simulink library "HY_General_Library"  (R2018b)
settings: Solver=ode45  StartTime=0.0  StopTime=10.0  RelTol=1e-3  EnableMultiTasking=on
undefined symbols (not defined in the file or in its folder): dT, Slope1, Slope2
libraries: simulink x63, $bdroot x4
(part 3 of 5)

== system HY_General_Library/Hysteresis_Blocks/HysteresisB ==
  OFF : Inport
  u : Inport  Port=2
  ON : Inport  Port=3
  RESET : Constant  Value=0  OutDataTypeStr=boolean
      settings: AttributesFormatString=%<OutDataTypeStr>
  Relational Operator : RelationalOperator  Operator=>  OutDataTypeStr=boolean  RndMeth=Nearest
  Relational Operator1 : RelationalOperator  Operator=<=  OutDataTypeStr=boolean  RndMeth=Nearest
  SET : Constant  OutDataTypeStr=boolean
      settings: AttributesFormatString=%<OutDataTypeStr>
  Switch : Switch  Criteria=u2 ~= 0  SaturateOnIntegerOverflow=on
  Switch1 : Switch  Criteria=u2 ~= 0  SaturateOnIntegerOverflow=on
  Unit Delay : UnitDelay  InitialCondition=InitialValue  SampleTime=-1
      settings: AttributesFormatString=Init: %<X0>
  y : Outport
  wires:
  RESET/1 -> Switch/1
  SET/1 -> Switch1/1
  Relational Operator/1 -> Switch/2
  Relational Operator1/1 -> Switch1/2
  Switch1/1 -> Switch/3
  Unit Delay/1 -> Switch1/3
  Switch/1 -> y/1, Unit Delay/1
  ON/1 -> Relational Operator1/2
  u/1 -> Relational Operator/1, Relational Operator1/1
  OFF/1 -> Relational Operator/2

== system HY_General_Library/Limit_Blocks/GrandientLimiter ==
  TargetValue : Inport  RequirementInfo={} %GIDa_f6d18a4e_084c_45e5_9882_4c3ecc41a03a
  BaseValue : Inport  RequirementInfo={} %GIDa_fa325680_5d49_4650_9e93_54c2fe60e26b  Port=2
  Reset : Inport  Port=3  OutDataTypeStr=boolean
  ResetValue : Inport  Port=4
  GrdtPos : Inport  RequirementInfo={} %GIDa_5e77dc31_cedd_4c5f_966e_ba8c10611931  Port=5
  GrdtNeg : Inport  RequirementInfo={} %GIDa_da933117_8913_4446_8ae4_767cc6412277  Port=6
  SampleTime : Inport  RequirementInfo={} %GIDa_02549e31_b069_4371_b83e_0eb5bce206e9  Port=7
  Abs1 : Abs
  Abs2 : Abs
  Gain1 : Gain  Gain=-1
  MinMax1 : MinMax  Function=max  Inputs=2
  MinMax2 : MinMax  Inputs=2
  Product : Product
  Product1 : Product
  Subtract : Sum  Inputs=+-
  Subtract1 : Sum
  Switch : Switch  Criteria=u2 ~= 0  SaturateOnIntegerOverflow=on
  GrdtLimdValue : Outport  RequirementInfo={} %GIDa_7967a4c3_b106_4517_b83e_55608d1226d7
  wires:
  MinMax2/1 -> MinMax1/2
  Gain1/1 -> MinMax1/1
  Abs2/1 -> Product/1
  MinMax1/1 -> Subtract1/1
  TargetValue/1 -> Subtract/1
  Abs1/1 -> Product1/2
  Product/1 -> Gain1/1
  SampleTime/1 -> Product1/1, Product/2
  Subtract/1 -> MinMax2/2
  Subtract1/1 -> Switch/3
  BaseValue/1 -> Subtract/2, Subtract1/2
  Product1/1 -> MinMax2/1
  GrdtPos/1 -> Abs1/1
  GrdtNeg/1 -> Abs2/1
  ResetValue/1 -> Switch/1
  Reset/1 -> Switch/2
  Switch/1 -> GrdtLimdValue/1

== system HY_General_Library/Limit_Blocks/LIMIT ==
  Max : Inport
  u : Inport  Port=2
  Min : Inport  Port=3
  Data Type Propagation : simulink/Signal Attributes/Data Type Propagation  PropDataType=fixdt(1, 16)  IfRefDouble=double  IfRefSingle=single  IsSigned=IsSigned1  NumBitsBase=NumBits1  NumBitsMult=1  NumBitsAdd=0  NumBitsAllowFinal=1:128  PropScaling=2^-10  ValuesUsedBestPrec=[5 -7]  SlopeBase=min([Slope1 Slope2])  SlopeMult=1  SlopeAdd=0  BiasBase=Bias1  BiasMult=1  BiasAdd=0
      settings: SourceProductName=Simulink  SourceProductBaseCode=SL
  Data Type Propagation1 : simulink/Signal Attributes/Data Type Propagation  PropDataType=fixdt(1, 16)  IfRefDouble=double  IfRefSingle=single  IsSigned=IsSigned1  NumBitsBase=NumBits1  NumBitsMult=1  NumBitsAdd=0  NumBitsAllowFinal=1:128  PropScaling=2^-10  ValuesUsedBestPrec=[5 -7]  SlopeBase=min([Slope1 Slope2])  SlopeMult=1  SlopeAdd=0  BiasBase=Bias1  BiasMult=1  BiasAdd=0
      settings: SourceProductName=Simulink  SourceProductBaseCode=SL
  MinMax : MinMax  Inputs=2  SaturateOnIntegerOverflow=on  InputSameDT=on
  MinMax1 : MinMax  Function=max  Inputs=2  OutDataTypeStr=Inherit: Inherit via back propagation  SaturateOnIntegerOverflow=on
  y : Outport  InitialOutput=0
  wires:
  MinMax/1 -> y/1, Data Type Propagation1/3
  MinMax1/1 -> MinMax/2, Data Type Propagation/3
  Min/1 -> MinMax1/2
  u/1 -> Data Type Propagation/2, Data Type Propagation/1, Data Type Propagation1/2, Data Type Propagation1/1, MinMax1/1
  Max/1 -> MinMax/1

== system HY_General_Library/Limit_Blocks/Limit_Flag ==
  Max : Inport
  u : Inport  Port=2
  Min : Inport  Port=3
  Data Type Propagation : simulink/Signal Attributes/Data Type Propagation  PropDataType=fixdt(1, 16)  IfRefDouble=double  IfRefSingle=single  IsSigned=IsSigned1  NumBitsBase=NumBits1  NumBitsMult=1  NumBitsAdd=0  NumBitsAllowFinal=1:128  PropScaling=2^-10  ValuesUsedBestPrec=[5 -7]  SlopeBase=min([Slope1 Slope2])  SlopeMult=1  SlopeAdd=0  BiasBase=Bias1  BiasMult=1  BiasAdd=0
      settings: SourceProductName=Simulink  SourceProductBaseCode=SL
  Data Type Propagation1 : simulink/Signal Attributes/Data Type Propagation  PropDataType=fixdt(1, 16)  IfRefDouble=double  IfRefSingle=single  IsSigned=IsSigned1  NumBitsBase=NumBits1  NumBitsMult=1  NumBitsAdd=0  NumBitsAllowFinal=1:128  PropScaling=2^-10  ValuesUsedBestPrec=[5 -7]  SlopeBase=min([Slope1 Slope2])  SlopeMult=1  SlopeAdd=0  BiasBase=Bias1  BiasMult=1  BiasAdd=0
      settings: SourceProductName=Simulink  SourceProductBaseCode=SL
  Logical Operator : Logic  OutDataTypeStr=boolean
  Logical Operator1 : Logic  Operator=NOT  Inputs=1  OutDataTypeStr=boolean
  MinMax : MinMax  Inputs=2  SaturateOnIntegerOverflow=on  InputSameDT=on
  MinMax1 : MinMax  Function=max  Inputs=2  OutDataTypeStr=Inherit: Inherit via back propagation  SaturateOnIntegerOverflow=on
  Relational Operator : RelationalOperator  Operator=>  OutDataTypeStr=boolean  RndMeth=Simplest  InputSameDT=on
  Relational Operator1 : RelationalOperator  Operator=<  OutDataTypeStr=boolean  RndMeth=Simplest  InputSameDT=on
  y : Outport  InitialOutput=0
  bMax : Outport  Port=2  InitialOutput=0
  bMin : Outport  Port=3  InitialOutput=0
  wires:
  Max/1 -> Relational Operator/2, MinMax/1
  u/1 -> MinMax1/1, Data Type Propagation1/1, Data Type Propagation1/2, Relational Operator1/1, Relational Operator/1, Data Type Propagation/2, Data Type Propagation/1
  Min/1 -> Relational Operator1/2, MinMax1/2
  MinMax1/1 -> Data Type Propagation/3, MinMax/2
  MinMax/1 -> Data Type Propagation1/3, y/1
  Logical Operator1/1 -> Logical Operator/1
  Relational Operator/1 -> Logical Operator1/1, bMax/1
  Logical Operator/1 -> bMin/1
  Relational Operator1/1 -> Logical Operator/2

== system HY_General_Library/Limit_Blocks/RateLimit_R ==
  u : Inport  RequirementInfo={} %GIDa_f6d18a4e_084c_45e5_9882_4c3ecc41a03a
  GrdtPos : Inport  RequirementInfo={} %GIDa_5e77dc31_cedd_4c5f_966e_ba8c10611931  Port=2
  GrdtNeg : Inport  RequirementInfo={} %GIDa_da933117_8913_4446_8ae4_767cc6412277  Port=3
  Reset : Inport  Port=4  OutDataTypeStr=boolean
  ResetVaule : Inport  Port=5
  dT : Inport  RequirementInfo={} %GIDa_02549e31_b069_4371_b83e_0eb5bce206e9  Port=6
  Constant : Constant  Value=0  OutDataTypeStr=boolean
      settings: AttributesFormatString=%<OutDataTypeStr>
  Constant1 : Constant  Value=0  OutDataTypeStr=Inherit: Inherit via back propagation
      settings: AttributesFormatString=%<OutDataTypeStr>
  Constant2 : Constant  Value=0  OutDataTypeStr=Inherit: Inherit via back propagation
      settings: AttributesFormatString=%<OutDataTypeStr>
  MinMax1 : MinMax  Function=max  Inputs=2  InputSameDT=on
  MinMax2 : MinMax  Inputs=2  InputSameDT=on
  MinMax3 : MinMax  Inputs=2  InputSameDT=on
  MinMax4 : MinMax  Function=max  Inputs=2  InputSameDT=on
  Product : Product
  Product1 : Product
  Subtract : Sum  Inputs=+-
  Subtract1 : Sum
  Switch : Switch  Criteria=u2 ~= 0  SaturateOnIntegerOverflow=on
      settings: AttributesFormatString=|
      | %<Criteria>
      | Threshold=%<Threshold>
  Switch1 : Switch  Criteria=u2 ~= 0  SaturateOnIntegerOverflow=on
      settings: AttributesFormatString=|
      | %<Criteria>
      | Threshold=%<Threshold>
  Unit Delay : UnitDelay  InitialCondition=1  SampleTime=-1
      settings: AttributesFormatString=<Initial=%<InitialCondition>>
  Unit Delay1 : UnitDelay  SampleTime=-1
      settings: AttributesFormatString=<Initial=%<InitialCondition>>
  y : Outport  RequirementInfo={} %GIDa_7967a4c3_b106_4517_b83e_55608d1226d7
  wires:
  Switch/1 -> Unit Delay1/1, y/1
  Reset/1 -> Switch/2
  ResetVaule/1 -> Switch/1
  Product1/1 -> MinMax3/1
  Subtract1/1 -> Switch1/3
  Subtract/1 -> MinMax1/2
  dT/1 -> Product1/1, Product/2
  Product/1 -> MinMax4/1
  GrdtPos/1 -> Product/1
  u/1 -> [u], Subtract/1
  MinMax2/1 -> Subtract1/1
  GrdtNeg/1 -> Product1/2
  MinMax4/1 -> MinMax2/1
  MinMax1/1 -> MinMax2/2
  Switch1/1 -> Switch/3
  Unit Delay/1 -> Switch1/2
  Constant/1 -> Unit Delay/1
  Unit Delay1/1 -> Subtract/2, Subtract1/2
  [u] -> Switch1/1
  Constant1/1 -> MinMax4/2
  Constant2/1 -> MinMax3/2
  MinMax3/1 -> MinMax1/1

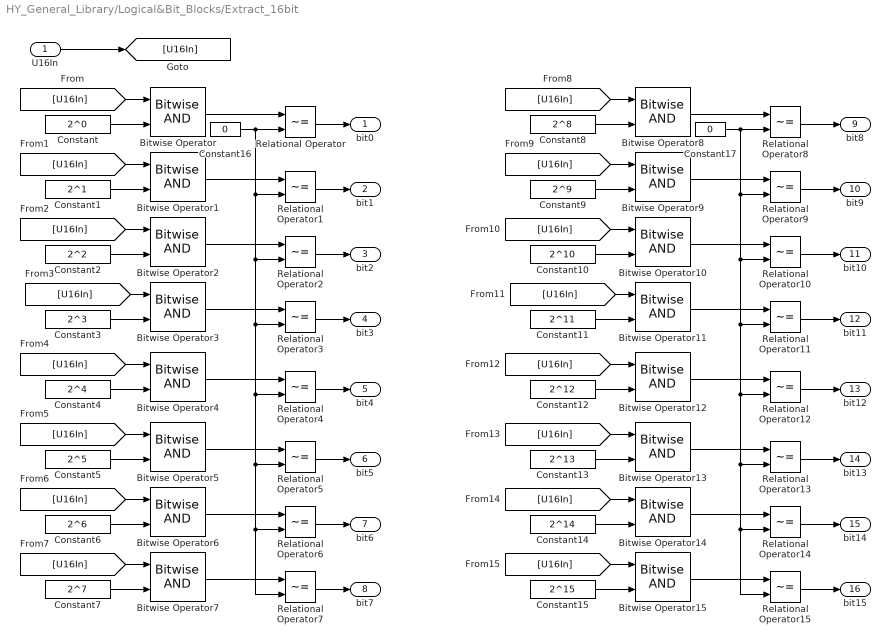
== system HY_General_Library/Logical&Bit_Blocks/Extract_16bit ==
  U16In : Inport
  Bitwise Operator{,1..15} (16 alike) : simulink/Logic and Bit Operations/Bitwise Operator  logicop=AND  UseBitMask=off  NumInputPorts=2  BitMask=bin2dec('11011001')  BitMaskRealWorld=Stored Integer
  Constant : Constant  Value=2^0  OutDataTypeStr=uint16
  Constant1 : Constant  Value=2^1  OutDataTypeStr=uint16
  Constant10 : Constant  Value=2^10  OutDataTypeStr=uint16
  Constant11 : Constant  Value=2^11  OutDataTypeStr=uint16
  Constant12 : Constant  Value=2^12  OutDataTypeStr=uint16
  Constant13 : Constant  Value=2^13  OutDataTypeStr=uint16
  Constant14 : Constant  Value=2^14  OutDataTypeStr=uint16
  Constant15 : Constant  Value=2^15  OutDataTypeStr=uint16
  Constant16 : Constant  Value=0  OutDataTypeStr=uint16
  Constant17 : Constant  Value=0  OutDataTypeStr=uint16
  Constant2 : Constant  Value=2^2  OutDataTypeStr=uint16
  Constant3 : Constant  Value=2^3  OutDataTypeStr=uint16
  Constant4 : Constant  Value=2^4  OutDataTypeStr=uint16
  Constant5 : Constant  Value=2^5  OutDataTypeStr=uint16
  Constant6 : Constant  Value=2^6  OutDataTypeStr=uint16
  Constant7 : Constant  Value=2^7  OutDataTypeStr=uint16
  Constant8 : Constant  Value=2^8  OutDataTypeStr=uint16
  Constant9 : Constant  Value=2^9  OutDataTypeStr=uint16
  Relational Operator{,1..15} (16 alike) : RelationalOperator  Operator=~=  OutDataTypeStr=boolean  RndMeth=Nearest
  bit0 : Outport
  bit1 : Outport  Port=2
  bit2 : Outport  Port=3
  bit3 : Outport  Port=4
  bit4 : Outport  Port=5
  bit5 : Outport  Port=6
  bit6 : Outport  Port=7
  bit7 : Outport  Port=8
  bit8 : Outport  Port=9
  bit9 : Outport  Port=10
  bit10 : Outport  Port=11
  bit11 : Outport  Port=12
  bit12 : Outport  Port=13
  bit13 : Outport  Port=14
  bit14 : Outport  Port=15
  bit15 : Outport  Port=16
  wires:
  U16In/1 -> [U16In]
  [U16In] -> Bitwise Operator/1
  Constant/1 -> Bitwise Operator/2
  [U16In] -> Bitwise Operator1/1
  Constant1/1 -> Bitwise Operator1/2
  [U16In] -> Bitwise Operator2/1
  Constant2/1 -> Bitwise Operator2/2
  [U16In] -> Bitwise Operator3/1
  Constant3/1 -> Bitwise Operator3/2
  [U16In] -> Bitwise Operator4/1
  Constant4/1 -> Bitwise Operator4/2
  [U16In] -> Bitwise Operator5/1
  Constant5/1 -> Bitwise Operator5/2
  [U16In] -> Bitwise Operator6/1
  Constant6/1 -> Bitwise Operator6/2
  [U16In] -> Bitwise Operator7/1
  Constant7/1 -> Bitwise Operator7/2
  Bitwise Operator1/1 -> Relational Operator1/1
  Bitwise Operator2/1 -> Relational Operator2/1
  Relational Operator2/1 -> bit2/1
  Relational Operator1/1 -> bit1/1
  Bitwise Operator3/1 -> Relational Operator3/1
  Relational Operator3/1 -> bit3/1
  Bitwise Operator4/1 -> Relational Operator4/1
  Relational Operator4/1 -> bit4/1
  Bitwise Operator5/1 -> Relational Operator5/1
  Relational Operator5/1 -> bit5/1
  Bitwise Operator6/1 -> Relational Operator6/1
  Relational Operator6/1 -> bit6/1
  Bitwise Operator7/1 -> Relational Operator7/1
  Relational Operator7/1 -> bit7/1
  [U16In] -> Bitwise Operator8/1
  Constant8/1 -> Bitwise Operator8/2
  [U16In] -> Bitwise Operator9/1
  Constant9/1 -> Bitwise Operator9/2
  [U16In] -> Bitwise Operator10/1
  Constant10/1 -> Bitwise Operator10/2
  [U16In] -> Bitwise Operator11/1
  Constant11/1 -> Bitwise Operator11/2
  [U16In] -> Bitwise Operator12/1
  Constant12/1 -> Bitwise Operator12/2
  [U16In] -> Bitwise Operator13/1
  Constant13/1 -> Bitwise Operator13/2
  [U16In] -> Bitwise Operator14/1
  Constant14/1 -> Bitwise Operator14/2
  [U16In] -> Bitwise Operator15/1
  Constant15/1 -> Bitwise Operator15/2
  Relational Operator10/1 -> bit10/1
  Relational Operator9/1 -> bit9/1
  Relational Operator8/1 -> bit8/1
  Relational Operator11/1 -> bit11/1
  Relational Operator12/1 -> bit12/1
  Relational Operator13/1 -> bit13/1
  Relational Operator14/1 -> bit14/1
  Relational Operator15/1 -> bit15/1
  Bitwise Operator/1 -> Relational Operator/1
  Relational Operator/1 -> bit0/1
  Constant16/1 -> Relational Operator1/2, Relational Operator2/2, Relational Operator3/2, Relational Operator4/2, Relational Operator5/2, Relational Operator7/2, Relational Operator6/2, Relational Operator/2
  Bitwise Operator9/1 -> Relational Operator9/1
  Bitwise Operator10/1 -> Relational Operator10/1
  Bitwise Operator11/1 -> Relational Operator11/1
  Bitwise Operator12/1 -> Relational Operator12/1
  Bitwise Operator13/1 -> Relational Operator13/1
  Bitwise Operator14/1 -> Relational Operator14/1
  Bitwise Operator15/1 -> Relational Operator15/1
  Bitwise Operator8/1 -> Relational Operator8/1
  Constant17/1 -> Relational Operator9/2, Relational Operator10/2, Relational Operator11/2, Relational Operator12/2, Relational Operator13/2, Relational Operator15/2, Relational Operator14/2, Relational Operator8/2

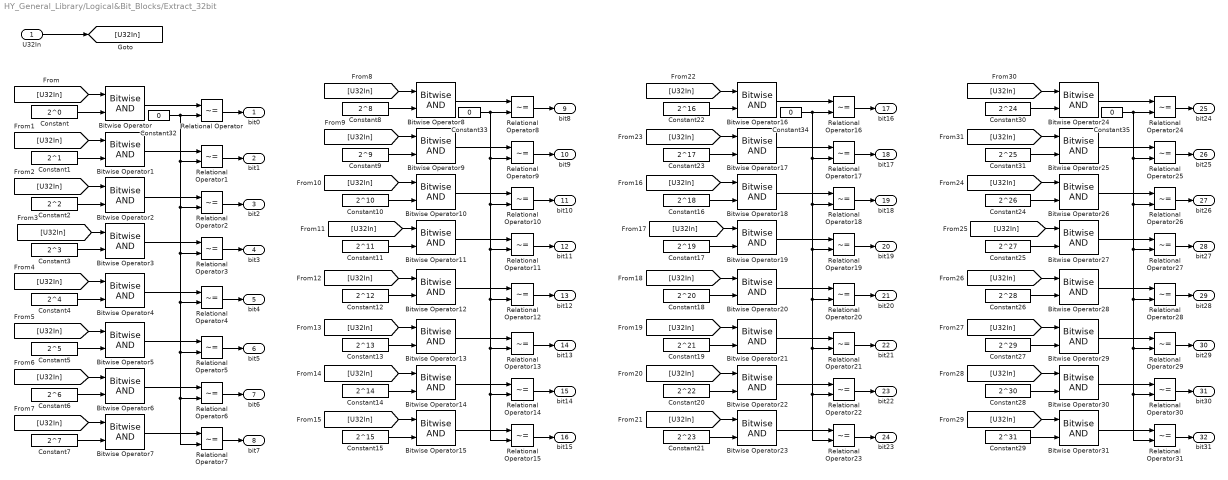
== system HY_General_Library/Logical&Bit_Blocks/Extract_32bit ==
  U32In : Inport
  Bitwise Operator{,1..31} (32 alike) : simulink/Logic and Bit Operations/Bitwise Operator  logicop=AND  UseBitMask=off  NumInputPorts=2  BitMask=bin2dec('11011001')  BitMaskRealWorld=Stored Integer
  Constant : Constant  Value=2^0  OutDataTypeStr=uint32
  Constant1 : Constant  Value=2^1  OutDataTypeStr=uint32
  Constant10 : Constant  Value=2^10  OutDataTypeStr=uint32
  Constant11 : Constant  Value=2^11  OutDataTypeStr=uint32
  Constant12 : Constant  Value=2^12  OutDataTypeStr=uint32
  Constant13 : Constant  Value=2^13  OutDataTypeStr=uint32
  Constant14 : Constant  Value=2^14  OutDataTypeStr=uint32
  Constant15 : Constant  Value=2^15  OutDataTypeStr=uint32
  Constant16 : Constant  Value=2^18  OutDataTypeStr=uint32
  Constant17 : Constant  Value=2^19  OutDataTypeStr=uint32
  Constant18 : Constant  Value=2^20  OutDataTypeStr=uint32
  Constant19 : Constant  Value=2^21  OutDataTypeStr=uint32
  Constant2 : Constant  Value=2^2  OutDataTypeStr=uint32
  Constant20 : Constant  Value=2^22  OutDataTypeStr=uint32
  Constant21 : Constant  Value=2^23  OutDataTypeStr=uint32
  Constant22 : Constant  Value=2^16  OutDataTypeStr=uint32
  Constant23 : Constant  Value=2^17  OutDataTypeStr=uint32
  Constant24 : Constant  Value=2^26  OutDataTypeStr=uint32
  Constant25 : Constant  Value=2^27  OutDataTypeStr=uint32
  Constant26 : Constant  Value=2^28  OutDataTypeStr=uint32
  Constant27 : Constant  Value=2^29  OutDataTypeStr=uint32
  Constant28 : Constant  Value=2^30  OutDataTypeStr=uint32
  Constant29 : Constant  Value=2^31  OutDataTypeStr=uint32
  Constant3 : Constant  Value=2^3  OutDataTypeStr=uint32
  Constant30 : Constant  Value=2^24  OutDataTypeStr=uint32
  Constant31 : Constant  Value=2^25  OutDataTypeStr=uint32
  Constant{32..35} (4 alike) : Constant  Value=0  OutDataTypeStr=uint32
  Constant4 : Constant  Value=2^4  OutDataTypeStr=uint32
  Constant5 : Constant  Value=2^5  OutDataTypeStr=uint32
  Constant6 : Constant  Value=2^6  OutDataTypeStr=uint32
  Constant7 : Constant  Value=2^7  OutDataTypeStr=uint32
  Constant8 : Constant  Value=2^8  OutDataTypeStr=uint32
  Constant9 : Constant  Value=2^9  OutDataTypeStr=uint32
  Relational Operator{,1..31} (32 alike) : RelationalOperator  Operator=~=  OutDataTypeStr=boolean  RndMeth=Nearest
  bit0 : Outport
  bit1 : Outport  Port=2
  bit2 : Outport  Port=3
  bit3 : Outport  Port=4
  bit4 : Outport  Port=5
  bit5 : Outport  Port=6
  bit6 : Outport  Port=7
  bit7 : Outport  Port=8
  bit8 : Outport  Port=9
  bit9 : Outport  Port=10
  bit10 : Outport  Port=11
  bit11 : Outport  Port=12
  bit12 : Outport  Port=13
  bit13 : Outport  Port=14
  bit14 : Outport  Port=15
  bit15 : Outport  Port=16
  bit16 : Outport  Port=17
  bit17 : Outport  Port=18
  bit18 : Outport  Port=19
  bit19 : Outport  Port=20
  bit20 : Outport  Port=21
  bit21 : Outport  Port=22
  bit22 : Outport  Port=23
  bit23 : Outport  Port=24
  bit24 : Outport  Port=25
  bit25 : Outport  Port=26
  bit26 : Outport  Port=27
  bit27 : Outport  Port=28
  bit28 : Outport  Port=29
  bit29 : Outport  Port=30
  bit30 : Outport  Port=31
  bit31 : Outport  Port=32
  wires:
  U32In/1 -> [U32In]
  [U32In] -> Bitwise Operator/1
  Constant/1 -> Bitwise Operator/2
  [U32In] -> Bitwise Operator1/1
  Constant1/1 -> Bitwise Operator1/2
  [U32In] -> Bitwise Operator2/1
  Constant2/1 -> Bitwise Operator2/2
  [U32In] -> Bitwise Operator3/1
  Constant3/1 -> Bitwise Operator3/2
  [U32In] -> Bitwise Operator4/1
  Constant4/1 -> Bitwise Operator4/2
  [U32In] -> Bitwise Operator5/1
  Constant5/1 -> Bitwise Operator5/2
  [U32In] -> Bitwise Operator6/1
  Constant6/1 -> Bitwise Operator6/2
  [U32In] -> Bitwise Operator7/1
  Constant7/1 -> Bitwise Operator7/2
  [U32In] -> Bitwise Operator8/1
  Constant8/1 -> Bitwise Operator8/2
  [U32In] -> Bitwise Operator9/1
  Constant9/1 -> Bitwise Operator9/2
  [U32In] -> Bitwise Operator10/1
  Constant10/1 -> Bitwise Operator10/2
  [U32In] -> Bitwise Operator11/1
  Constant11/1 -> Bitwise Operator11/2
  [U32In] -> Bitwise Operator12/1
  Constant12/1 -> Bitwise Operator12/2
  [U32In] -> Bitwise Operator13/1
  Constant13/1 -> Bitwise Operator13/2
  [U32In] -> Bitwise Operator14/1
  Constant14/1 -> Bitwise Operator14/2
  [U32In] -> Bitwise Operator15/1
  Constant15/1 -> Bitwise Operator15/2
  [U32In] -> Bitwise Operator16/1
  Constant22/1 -> Bitwise Operator16/2
  [U32In] -> Bitwise Operator17/1
  Constant23/1 -> Bitwise Operator17/2
  [U32In] -> Bitwise Operator18/1
  Constant16/1 -> Bitwise Operator18/2
  [U32In] -> Bitwise Operator19/1
  Constant17/1 -> Bitwise Operator19/2
  [U32In] -> Bitwise Operator20/1
  Constant18/1 -> Bitwise Operator20/2
  [U32In] -> Bitwise Operator21/1
  Constant19/1 -> Bitwise Operator21/2
  [U32In] -> Bitwise Operator22/1
  Constant20/1 -> Bitwise Operator22/2
  [U32In] -> Bitwise Operator23/1
  Constant21/1 -> Bitwise Operator23/2
  [U32In] -> Bitwise Operator24/1
  Constant30/1 -> Bitwise Operator24/2
  [U32In] -> Bitwise Operator25/1
  Constant31/1 -> Bitwise Operator25/2
  [U32In] -> Bitwise Operator26/1
  Constant24/1 -> Bitwise Operator26/2
  [U32In] -> Bitwise Operator27/1
  Constant25/1 -> Bitwise Operator27/2
  [U32In] -> Bitwise Operator28/1
  Constant26/1 -> Bitwise Operator28/2
  [U32In] -> Bitwise Operator29/1
  Constant27/1 -> Bitwise Operator29/2
  [U32In] -> Bitwise Operator30/1
  Constant28/1 -> Bitwise Operator30/2
  [U32In] -> Bitwise Operator31/1
  Constant29/1 -> Bitwise Operator31/2
  Bitwise Operator1/1 -> Relational Operator1/1
  Bitwise Operator2/1 -> Relational Operator2/1
  Relational Operator2/1 -> bit2/1
  Relational Operator1/1 -> bit1/1
  Bitwise Operator3/1 -> Relational Operator3/1
  Relational Operator3/1 -> bit3/1
  Bitwise Operator4/1 -> Relational Operator4/1
  Relational Operator4/1 -> bit4/1
  Bitwise Operator5/1 -> Relational Operator5/1
  Relational Operator5/1 -> bit5/1
  Bitwise Operator6/1 -> Relational Operator6/1
  Relational Operator6/1 -> bit6/1
  Bitwise Operator7/1 -> Relational Operator7/1
  Relational Operator7/1 -> bit7/1
  Bitwise Operator/1 -> Relational Operator/1
  Relational Operator/1 -> bit0/1
  Constant32/1 -> Relational Operator1/2, Relational Operator2/2, Relational Operator3/2, Relational Operator4/2, Relational Operator5/2, Relational Operator7/2, Relational Operator6/2, Relational Operator/2
  Bitwise Operator9/1 -> Relational Operator9/1
  Bitwise Operator10/1 -> Relational Operator10/1
  Relational Operator10/1 -> bit10/1
  Relational Operator9/1 -> bit9/1
  Bitwise Operator11/1 -> Relational Operator11/1
  Relational Operator11/1 -> bit11/1
  Bitwise Operator12/1 -> Relational Operator12/1
  Relational Operator12/1 -> bit12/1
  Bitwise Operator13/1 -> Relational Operator13/1
  Relational Operator13/1 -> bit13/1
  Bitwise Operator14/1 -> Relational Operator14/1
  Relational Operator14/1 -> bit14/1
  Bitwise Operator15/1 -> Relational Operator15/1
  Relational Operator15/1 -> bit15/1
  Bitwise Operator8/1 -> Relational Operator8/1
  Relational Operator8/1 -> bit8/1
  Constant33/1 -> Relational Operator9/2, Relational Operator10/2, Relational Operator11/2, Relational Operator12/2, Relational Operator13/2, Relational Operator15/2, Relational Operator14/2, Relational Operator8/2
  Bitwise Operator17/1 -> Relational Operator17/1
  Bitwise Operator18/1 -> Relational Operator18/1
  Relational Operator18/1 -> bit18/1
  Relational Operator17/1 -> bit17/1
  Bitwise Operator19/1 -> Relational Operator19/1
  Relational Operator19/1 -> bit19/1
  Bitwise Operator20/1 -> Relational Operator20/1
  Relational Operator20/1 -> bit20/1
  Bitwise Operator21/1 -> Relational Operator21/1
  Relational Operator21/1 -> bit21/1
  Bitwise Operator22/1 -> Relational Operator22/1
  Relational Operator22/1 -> bit22/1
  Bitwise Operator23/1 -> Relational Operator23/1
  Relational Operator23/1 -> bit23/1
  Bitwise Operator16/1 -> Relational Operator16/1
  Relational Operator16/1 -> bit16/1
  Constant34/1 -> Relational Operator17/2, Relational Operator18/2, Relational Operator19/2, Relational Operator20/2, Relational Operator21/2, Relational Operator23/2, Relational Operator22/2, Relational Operator16/2
  Bitwise Operator25/1 -> Relational Operator25/1
  Bitwise Operator26/1 -> Relational Operator26/1
  Relational Operator26/1 -> bit26/1
  Relational Operator25/1 -> bit25/1
  Bitwise Operator27/1 -> Relational Operator27/1
  Relational Operator27/1 -> bit27/1
  Bitwise Operator28/1 -> Relational Operator28/1
  Relational Operator28/1 -> bit28/1
  Bitwise Operator29/1 -> Relational Operator29/1
  Relational Operator29/1 -> bit29/1
  Bitwise Operator30/1 -> Relational Operator30/1
  Relational Operator30/1 -> bit30/1
  Bitwise Operator31/1 -> Relational Operator31/1
  Relational Operator31/1 -> bit31/1
  Bitwise Operator24/1 -> Relational Operator24/1
  Relational Operator24/1 -> bit24/1
  Constant35/1 -> Relational Operator25/2, Relational Operator26/2, Relational Operator27/2, Relational Operator28/2, Relational Operator29/2, Relational Operator31/2, Relational Operator30/2, Relational Operator24/2

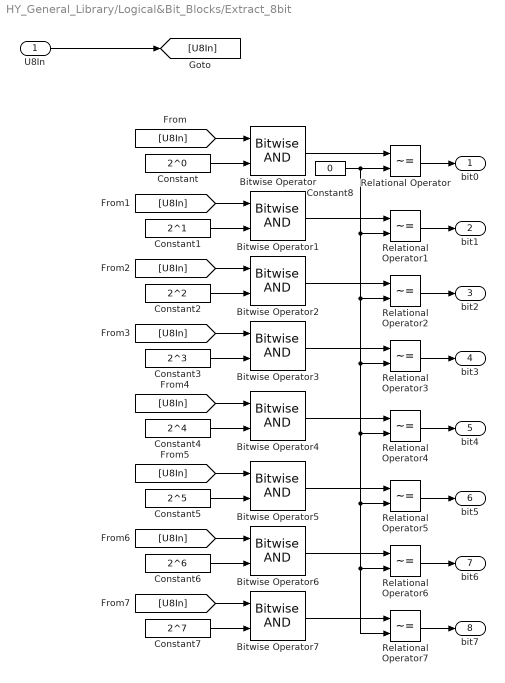
== system HY_General_Library/Logical&Bit_Blocks/Extract_8bit ==
  U8In : Inport
  Bitwise Operator{,1..7} (8 alike) : simulink/Logic and Bit Operations/Bitwise Operator  logicop=AND  UseBitMask=off  NumInputPorts=2  BitMask=bin2dec('11011001')  BitMaskRealWorld=Stored Integer
  Constant : Constant  Value=2^0  OutDataTypeStr=uint8
  Constant1 : Constant  Value=2^1  OutDataTypeStr=uint8
  Constant2 : Constant  Value=2^2  OutDataTypeStr=uint8
  Constant3 : Constant  Value=2^3  OutDataTypeStr=uint8
  Constant4 : Constant  Value=2^4  OutDataTypeStr=uint8
  Constant5 : Constant  Value=2^5  OutDataTypeStr=uint8
  Constant6 : Constant  Value=2^6  OutDataTypeStr=uint8
  Constant7 : Constant  Value=2^7  OutDataTypeStr=uint8
  Constant8 : Constant  Value=0  OutDataTypeStr=uint8
  Relational Operator{,1..7} (8 alike) : RelationalOperator  Operator=~=  OutDataTypeStr=boolean  RndMeth=Nearest
  bit0 : Outport
  bit1 : Outport  Port=2
  bit2 : Outport  Port=3
  bit3 : Outport  Port=4
  bit4 : Outport  Port=5
  bit5 : Outport  Port=6
  bit6 : Outport  Port=7
  bit7 : Outport  Port=8
  wires:
  Constant/1 -> Bitwise Operator/2
  Constant1/1 -> Bitwise Operator1/2
  Constant2/1 -> Bitwise Operator2/2
  Constant3/1 -> Bitwise Operator3/2
  Constant4/1 -> Bitwise Operator4/2
  Constant5/1 -> Bitwise Operator5/2
  Constant6/1 -> Bitwise Operator6/2
  Constant7/1 -> Bitwise Operator7/2
  Bitwise Operator/1 -> Relational Operator/1
  Bitwise Operator1/1 -> Relational Operator1/1
  Bitwise Operator2/1 -> Relational Operator2/1
  Relational Operator2/1 -> bit2/1
  Relational Operator1/1 -> bit1/1
  Relational Operator/1 -> bit0/1
  Bitwise Operator3/1 -> Relational Operator3/1
  Relational Operator3/1 -> bit3/1
  Bitwise Operator4/1 -> Relational Operator4/1
  Relational Operator4/1 -> bit4/1
  Bitwise Operator5/1 -> Relational Operator5/1
  Relational Operator5/1 -> bit5/1
  Bitwise Operator6/1 -> Relational Operator6/1
  Relational Operator6/1 -> bit6/1
  Bitwise Operator7/1 -> Relational Operator7/1
  Relational Operator7/1 -> bit7/1
  Constant8/1 -> Relational Operator7/2, Relational Operator6/2, Relational Operator5/2, Relational Operator4/2, Relational Operator3/2, Relational Operator2/2, Relational Operator1/2, Relational Operator/2
  [U8In] -> Bitwise Operator/1
  U8In/1 -> [U8In]
  [U8In] -> Bitwise Operator1/1
  [U8In] -> Bitwise Operator2/1
  [U8In] -> Bitwise Operator3/1
  [U8In] -> Bitwise Operator4/1
  [U8In] -> Bitwise Operator5/1
  [U8In] -> Bitwise Operator6/1
  [U8In] -> Bitwise Operator7/1

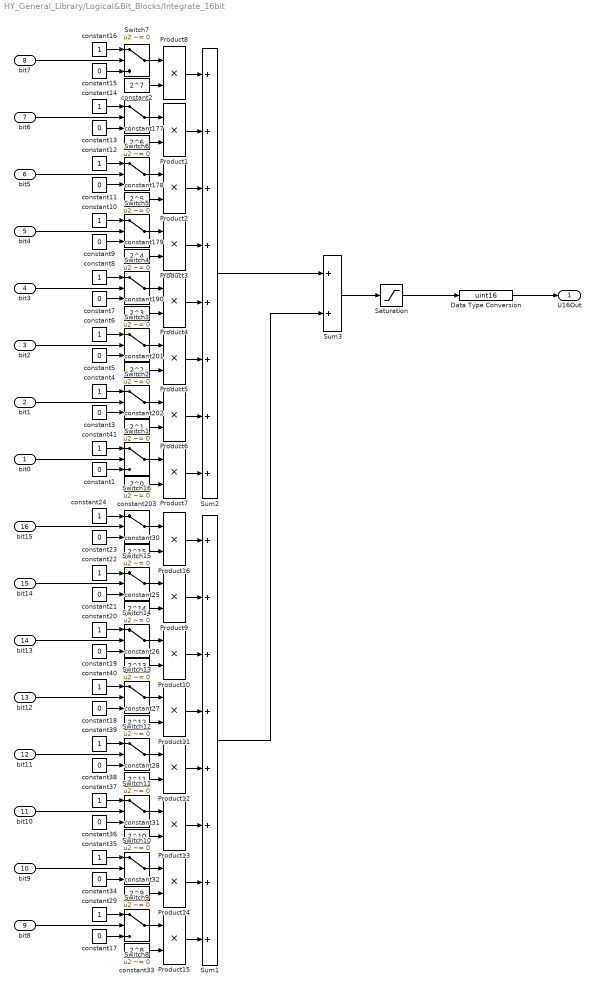
== system HY_General_Library/Logical&Bit_Blocks/Integrate_16bit ==
  bit0 : Inport
  bit1 : Inport  Port=2
  bit2 : Inport  Port=3
  bit3 : Inport  Port=4
  bit4 : Inport  Port=5
  bit5 : Inport  Port=6
  bit6 : Inport  Port=7
  bit7 : Inport  Port=8
  bit8 : Inport  Port=9
  bit9 : Inport  Port=10
  bit10 : Inport  Port=11
  bit11 : Inport  Port=12
  bit12 : Inport  Port=13
  bit13 : Inport  Port=14
  bit14 : Inport  Port=15
  bit15 : Inport  Port=16
  Data Type Conversion : DataTypeConversion  OutDataTypeStr=uint16
  Product{1..16} (16 alike) : Product  SaturateOnIntegerOverflow=on  InputSameDT=on  OutDataTypeStr=Inherit: Same as first input
  Saturation : Saturate  UpperLimit=65535  LowerLimit=0
      settings: AttributesFormatString=%<LowerLimit> - %<UpperLimit>
  Sum1 : Sum  Inputs=8  SaturateOnIntegerOverflow=on  InputSameDT=on  OutDataTypeStr=Inherit: Same as first input
  Sum2 : Sum  Inputs=8  SaturateOnIntegerOverflow=on  InputSameDT=on  OutDataTypeStr=Inherit: Same as first input
  Sum3 : Sum  Inputs=2  SaturateOnIntegerOverflow=on  InputSameDT=on  OutDataTypeStr=Inherit: Same as first input
  Switch{1..16} (16 alike) : Switch  Criteria=u2 ~= 0  SaturateOnIntegerOverflow=on  InputSameDT=on
  constant{1,3,5,7,9,11,13,15,17..19,21,23,34,36,38} (16 alike) : Constant  Value=0  OutDataTypeStr=uint16
  constant{4,6,8,10,12,14,16,20,22,24,29,35,37,39..41} (16 alike) : Constant  OutDataTypeStr=uint16
  constant177 : Constant  Value=2^6  OutDataTypeStr=uint16
  constant178 : Constant  Value=2^5  OutDataTypeStr=uint16
  constant179 : Constant  Value=2^4  OutDataTypeStr=uint16
  constant190 : Constant  Value=2^3  OutDataTypeStr=uint16
  constant2 : Constant  Value=2^7  OutDataTypeStr=uint16
  constant201 : Constant  Value=2^2  OutDataTypeStr=uint16
  constant202 : Constant  Value=2^1  OutDataTypeStr=uint16
  constant203 : Constant  Value=2^0  OutDataTypeStr=uint16
  constant25 : Constant  Value=2^14  OutDataTypeStr=uint16
  constant26 : Constant  Value=2^13  OutDataTypeStr=uint16
  constant27 : Constant  Value=2^12  OutDataTypeStr=uint16
  constant28 : Constant  Value=2^11  OutDataTypeStr=uint16
  constant30 : Constant  Value=2^15  OutDataTypeStr=uint16
  constant31 : Constant  Value=2^10  OutDataTypeStr=uint16
  constant32 : Constant  Value=2^9  OutDataTypeStr=uint16
  constant33 : Constant  Value=2^8  OutDataTypeStr=uint16
  U16Out : Outport
  wires:
  Switch7/1 -> Product8/1
  constant2/1 -> Product8/2
  Product8/1 -> Sum2/1
  Switch16/1 -> Product7/1
  Switch6/1 -> Product1/1
  constant177/1 -> Product1/2
  constant178/1 -> Product2/2
  constant179/1 -> Product3/2
  constant190/1 -> Product4/2
  constant201/1 -> Product5/2
  constant202/1 -> Product6/2
  constant203/1 -> Product7/2
  Product1/1 -> Sum2/2
  Product2/1 -> Sum2/3
  Product3/1 -> Sum2/4
  Product4/1 -> Sum2/5
  Product5/1 -> Sum2/6
  Product6/1 -> Sum2/7
  Product7/1 -> Sum2/8
  constant30/1 -> Product16/2
  Product16/1 -> Sum1/1
  constant25/1 -> Product9/2
  constant26/1 -> Product10/2
  constant27/1 -> Product11/2
  constant28/1 -> Product12/2
  constant31/1 -> Product13/2
  constant32/1 -> Product14/2
  constant33/1 -> Product15/2
  Product9/1 -> Sum1/2
  Product10/1 -> Sum1/3
  Product11/1 -> Sum1/4
  Product12/1 -> Sum1/5
  Product13/1 -> Sum1/6
  Product14/1 -> Sum1/7
  Product15/1 -> Sum1/8
  Sum1/1 -> Sum3/2
  Sum2/1 -> Sum3/1
  Sum3/1 -> Saturation/1
  constant15/1 -> Switch7/3
  constant16/1 -> Switch7/1
  bit7/1 -> Switch7/2
  constant13/1 -> Switch6/3
  constant14/1 -> Switch6/1
  bit6/1 -> Switch6/2
  constant11/1 -> Switch5/3
  constant12/1 -> Switch5/1
  bit5/1 -> Switch5/2
  Switch5/1 -> Product2/1
  constant9/1 -> Switch4/3
  constant10/1 -> Switch4/1
  bit4/1 -> Switch4/2
  Switch4/1 -> Product3/1
  constant7/1 -> Switch3/3
  constant8/1 -> Switch3/1
  bit3/1 -> Switch3/2
  Switch3/1 -> Product4/1
  constant5/1 -> Switch2/3
  constant6/1 -> Switch2/1
  bit2/1 -> Switch2/2
  Switch2/1 -> Product5/1
  constant3/1 -> Switch1/3
  constant4/1 -> Switch1/1
  bit1/1 -> Switch1/2
  Switch1/1 -> Product6/1
  constant1/1 -> Switch16/3
  constant41/1 -> Switch16/1
  bit0/1 -> Switch16/2
  constant23/1 -> Switch15/3
  constant24/1 -> Switch15/1
  bit15/1 -> Switch15/2
  Switch15/1 -> Product16/1
  constant21/1 -> Switch14/3
  constant22/1 -> Switch14/1
  bit14/1 -> Switch14/2
  Switch14/1 -> Product9/1
  constant19/1 -> Switch13/3
  constant20/1 -> Switch13/1
  bit13/1 -> Switch13/2
  Switch13/1 -> Product10/1
  constant18/1 -> Switch12/3
  constant40/1 -> Switch12/1
  bit12/1 -> Switch12/2
  Switch12/1 -> Product11/1
  constant38/1 -> Switch11/3
  constant39/1 -> Switch11/1
  bit11/1 -> Switch11/2
  Switch11/1 -> Product12/1
  constant36/1 -> Switch10/3
  constant37/1 -> Switch10/1
  bit10/1 -> Switch10/2
  Switch10/1 -> Product13/1
  constant34/1 -> Switch9/3
  constant35/1 -> Switch9/1
  bit9/1 -> Switch9/2
  Switch9/1 -> Product14/1
  constant17/1 -> Switch8/3
  constant29/1 -> Switch8/1
  bit8/1 -> Switch8/2
  Switch8/1 -> Product15/1
  Saturation/1 -> Data Type Conversion/1
  Data Type Conversion/1 -> U16Out/1

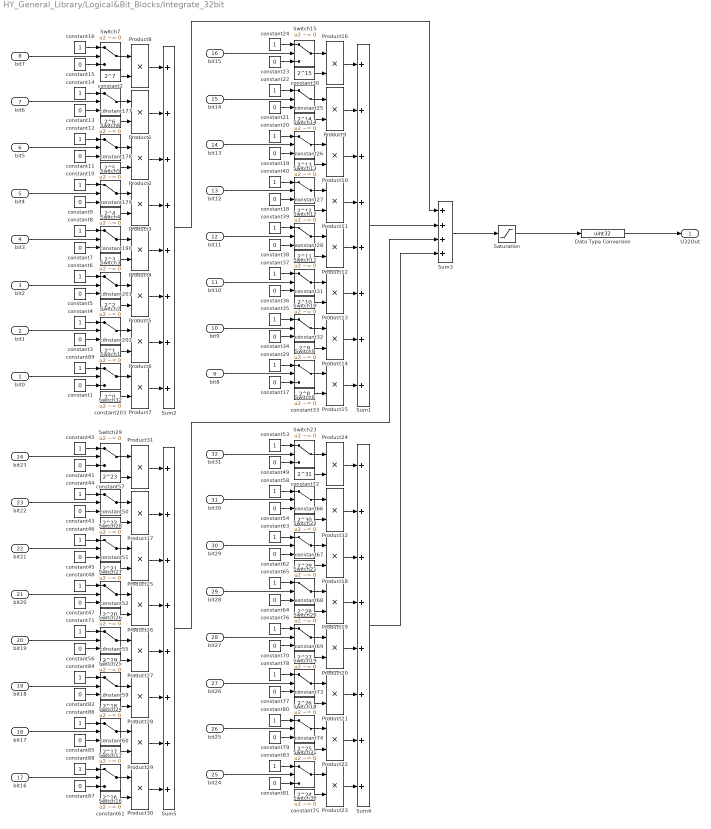
== system HY_General_Library/Logical&Bit_Blocks/Integrate_32bit ==
  bit0 : Inport
  bit1 : Inport  Port=2
  bit2 : Inport  Port=3
  bit3 : Inport  Port=4
  bit4 : Inport  Port=5
  bit5 : Inport  Port=6
  bit6 : Inport  Port=7
  bit7 : Inport  Port=8
  bit8 : Inport  Port=9
  bit9 : Inport  Port=10
  bit10 : Inport  Port=11
  bit11 : Inport  Port=12
  bit12 : Inport  Port=13
  bit13 : Inport  Port=14
  bit14 : Inport  Port=15
  bit15 : Inport  Port=16
  bit16 : Inport  Port=17
  bit17 : Inport  Port=18
  bit18 : Inport  Port=19
  bit19 : Inport  Port=20
  bit20 : Inport  Port=21
  bit21 : Inport  Port=22
  bit22 : Inport  Port=23
  bit23 : Inport  Port=24
  bit24 : Inport  Port=25
  bit25 : Inport  Port=26
  bit26 : Inport  Port=27
  bit27 : Inport  Port=28
  bit28 : Inport  Port=29
  bit29 : Inport  Port=30
  bit30 : Inport  Port=31
  bit31 : Inport  Port=32
  Data Type Conversion : DataTypeConversion  OutDataTypeStr=uint32
  Product{1..32} (32 alike) : Product  SaturateOnIntegerOverflow=on  InputSameDT=on  OutDataTypeStr=Inherit: Same as first input
  Saturation : Saturate  UpperLimit=4294967295  LowerLimit=0
      settings: AttributesFormatString=%<LowerLimit> - %<UpperLimit>
  Sum{1..2,4..5} (4 alike) : Sum  Inputs=8  SaturateOnIntegerOverflow=on  InputSameDT=on  OutDataTypeStr=Inherit: Same as first input
  Sum3 : Sum  Inputs=4  SaturateOnIntegerOverflow=on  InputSameDT=on  OutDataTypeStr=Inherit: Same as first input
  Switch{1..32} (32 alike) : Switch  Criteria=u2 ~= 0  SaturateOnIntegerOverflow=on  InputSameDT=on
  constant{1,3,5,7,9,11,13,15,17..19,21,23,34,36,38,41,43,45,47,49,54,56,62,64,70,77,79,81..82,85,87} (32 alike) : Constant  Value=0  OutDataTypeStr=uint32
  constant{4,6,8,10,12,14,16,20,22,24,29,35,37,39..40,42,44,46,48,53,58,63,65,71,76,78,80,83..84,86,88..89} (32 alike) : Constant  OutDataTypeStr=uint32
  constant177 : Constant  Value=2^6  OutDataTypeStr=uint32
  constant178 : Constant  Value=2^5  OutDataTypeStr=uint32
  constant179 : Constant  Value=2^4  OutDataTypeStr=uint32
  constant190 : Constant  Value=2^3  OutDataTypeStr=uint32
  constant2 : Constant  Value=2^7  OutDataTypeStr=uint32
  constant201 : Constant  Value=2^2  OutDataTypeStr=uint32
  constant202 : Constant  Value=2^1  OutDataTypeStr=uint32
  constant203 : Constant  Value=2^0  OutDataTypeStr=uint32
  constant25 : Constant  Value=2^14  OutDataTypeStr=uint32
  constant26 : Constant  Value=2^13  OutDataTypeStr=uint32
  constant27 : Constant  Value=2^12  OutDataTypeStr=uint32
  constant28 : Constant  Value=2^11  OutDataTypeStr=uint32
  constant30 : Constant  Value=2^15  OutDataTypeStr=uint32
  constant31 : Constant  Value=2^10  OutDataTypeStr=uint32
  constant32 : Constant  Value=2^9  OutDataTypeStr=uint32
  constant33 : Constant  Value=2^8  OutDataTypeStr=uint32
  constant50 : Constant  Value=2^22  OutDataTypeStr=uint32
  constant51 : Constant  Value=2^21  OutDataTypeStr=uint32
  constant52 : Constant  Value=2^20  OutDataTypeStr=uint32
  constant55 : Constant  Value=2^19  OutDataTypeStr=uint32
  constant57 : Constant  Value=2^23  OutDataTypeStr=uint32
  constant59 : Constant  Value=2^18  OutDataTypeStr=uint32
  constant60 : Constant  Value=2^17  OutDataTypeStr=uint32
  constant61 : Constant  Value=2^16  OutDataTypeStr=uint32
  constant66 : Constant  Value=2^30  OutDataTypeStr=uint32
  constant67 : Constant  Value=2^29  OutDataTypeStr=uint32
  constant68 : Constant  Value=2^28  OutDataTypeStr=uint32
  constant69 : Constant  Value=2^27  OutDataTypeStr=uint32
  constant72 : Constant  Value=2^31  OutDataTypeStr=uint32
  constant73 : Constant  Value=2^26  OutDataTypeStr=uint32
  constant74 : Constant  Value=2^25  OutDataTypeStr=uint32
  constant75 : Constant  Value=2^24  OutDataTypeStr=uint32
  U32Out : Outport
  wires:
  Sum3/1 -> Saturation/1
  Sum2/1 -> Sum3/1
  Sum1/1 -> Sum3/2
  Product15/1 -> Sum1/8
  Product14/1 -> Sum1/7
  Product13/1 -> Sum1/6
  Product12/1 -> Sum1/5
  Product11/1 -> Sum1/4
  Product10/1 -> Sum1/3
  Product9/1 -> Sum1/2
  constant33/1 -> Product15/2
  constant32/1 -> Product14/2
  constant31/1 -> Product13/2
  constant28/1 -> Product12/2
  constant27/1 -> Product11/2
  constant26/1 -> Product10/2
  constant25/1 -> Product9/2
  Switch8/1 -> Product15/1
  Product16/1 -> Sum1/1
  constant30/1 -> Product16/2
  Switch15/1 -> Product16/1
  Product7/1 -> Sum2/8
  Product6/1 -> Sum2/7
  Product5/1 -> Sum2/6
  Product4/1 -> Sum2/5
  Product3/1 -> Sum2/4
  Product2/1 -> Sum2/3
  Product1/1 -> Sum2/2
  constant203/1 -> Product7/2
  constant202/1 -> Product6/2
  constant201/1 -> Product5/2
  constant190/1 -> Product4/2
  constant179/1 -> Product3/2
  constant178/1 -> Product2/2
  constant177/1 -> Product1/2
  Switch6/1 -> Product1/1
  Product8/1 -> Sum2/1
  constant2/1 -> Product8/2
  Switch7/1 -> Product8/1
  Sum5/1 -> Sum3/3
  Product23/1 -> Sum4/8
  Product22/1 -> Sum4/7
  Product21/1 -> Sum4/6
  Product20/1 -> Sum4/5
  Product19/1 -> Sum4/4
  Product18/1 -> Sum4/3
  Product32/1 -> Sum4/2
  constant75/1 -> Product23/2
  constant74/1 -> Product22/2
  constant73/1 -> Product21/2
  constant69/1 -> Product20/2
  constant68/1 -> Product19/2
  constant67/1 -> Product18/2
  constant66/1 -> Product32/2
  Switch22/1 -> Product32/1
  Product24/1 -> Sum4/1
  constant72/1 -> Product24/2
  Switch23/1 -> Product24/1
  Product30/1 -> Sum5/8
  Product29/1 -> Sum5/7
  Product28/1 -> Sum5/6
  Product27/1 -> Sum5/5
  Product26/1 -> Sum5/4
  Product25/1 -> Sum5/3
  Product17/1 -> Sum5/2
  constant61/1 -> Product30/2
  constant60/1 -> Product29/2
  constant59/1 -> Product28/2
  constant55/1 -> Product27/2
  constant52/1 -> Product26/2
  constant51/1 -> Product25/2
  constant50/1 -> Product17/2
  Switch16/1 -> Product30/1
  Product31/1 -> Sum5/1
  constant57/1 -> Product31/2
  Switch29/1 -> Product31/1
  Sum4/1 -> Sum3/4
  constant15/1 -> Switch7/3
  constant16/1 -> Switch7/1
  constant13/1 -> Switch6/3
  constant14/1 -> Switch6/1
  bit7/1 -> Switch7/2
  constant11/1 -> Switch5/3
  constant12/1 -> Switch5/1
  Switch5/1 -> Product2/1
  bit6/1 -> Switch6/2
  bit5/1 -> Switch5/2
  constant9/1 -> Switch4/3
  constant10/1 -> Switch4/1
  Switch4/1 -> Product3/1
  bit4/1 -> Switch4/2
  constant7/1 -> Switch3/3
  constant8/1 -> Switch3/1
  Switch3/1 -> Product4/1
  bit3/1 -> Switch3/2
  constant5/1 -> Switch2/3
  constant6/1 -> Switch2/1
  Switch2/1 -> Product5/1
  bit2/1 -> Switch2/2
  constant3/1 -> Switch1/3
  constant4/1 -> Switch1/1
  Switch1/1 -> Product6/1
  bit1/1 -> Switch1/2
  constant1/1 -> Switch32/3
  constant89/1 -> Switch32/1
  Switch32/1 -> Product7/1
  bit0/1 -> Switch32/2
  constant23/1 -> Switch15/3
  constant24/1 -> Switch15/1
  bit15/1 -> Switch15/2
  constant21/1 -> Switch14/3
  constant22/1 -> Switch14/1
  Switch14/1 -> Product9/1
  bit14/1 -> Switch14/2
  constant19/1 -> Switch13/3
  constant20/1 -> Switch13/1
  Switch13/1 -> Product10/1
  bit13/1 -> Switch13/2
  constant18/1 -> Switch12/3
  constant40/1 -> Switch12/1
  Switch12/1 -> Product11/1
  bit12/1 -> Switch12/2
  constant38/1 -> Switch11/3
  constant39/1 -> Switch11/1
  Switch11/1 -> Product12/1
  bit11/1 -> Switch11/2
  constant36/1 -> Switch10/3
  constant37/1 -> Switch10/1
  Switch10/1 -> Product13/1
  bit10/1 -> Switch10/2
  constant34/1 -> Switch9/3
  constant35/1 -> Switch9/1
  Switch9/1 -> Product14/1
  bit9/1 -> Switch9/2
  constant17/1 -> Switch8/3
  constant29/1 -> Switch8/1
  bit8/1 -> Switch8/2
  constant41/1 -> Switch29/3
  constant42/1 -> Switch29/1
  bit23/1 -> Switch29/2
  constant43/1 -> Switch28/3
  constant44/1 -> Switch28/1
  Switch28/1 -> Product17/1
  bit22/1 -> Switch28/2
  constant45/1 -> Switch27/3
  constant46/1 -> Switch27/1
  Switch27/1 -> Product25/1
  bit21/1 -> Switch27/2
  constant47/1 -> Switch26/3
  constant48/1 -> Switch26/1
  bit20/1 -> Switch26/2
  Switch26/1 -> Product26/1
  constant56/1 -> Switch25/3
  constant71/1 -> Switch25/1
  Switch25/1 -> Product27/1
  bit19/1 -> Switch25/2
  constant82/1 -> Switch24/3
  constant84/1 -> Switch24/1
  Switch24/1 -> Product28/1
  bit18/1 -> Switch24/2
  constant85/1 -> Switch17/3
  constant86/1 -> Switch17/1
  Switch17/1 -> Product29/1
  bit17/1 -> Switch17/2
  constant87/1 -> Switch16/3
  constant88/1 -> Switch16/1
  bit16/1 -> Switch16/2
  constant49/1 -> Switch23/3
  constant53/1 -> Switch23/1
  bit31/1 -> Switch23/2
  constant54/1 -> Switch22/3
  constant58/1 -> Switch22/1
  bit30/1 -> Switch22/2
  constant62/1 -> Switch21/3
  constant63/1 -> Switch21/1
  Switch21/1 -> Product18/1
  bit29/1 -> Switch21/2
  constant64/1 -> Switch20/3
  constant65/1 -> Switch20/1
  Switch20/1 -> Product19/1
  bit28/1 -> Switch20/2
  constant70/1 -> Switch19/3
  constant76/1 -> Switch19/1
  Switch19/1 -> Product20/1
  bit27/1 -> Switch19/2
  constant77/1 -> Switch18/3
  constant78/1 -> Switch18/1
  Switch18/1 -> Product21/1
  bit26/1 -> Switch18/2
  constant79/1 -> Switch31/3
  constant80/1 -> Switch31/1
  Switch31/1 -> Product22/1
  bit25/1 -> Switch31/2
  constant81/1 -> Switch30/3
  constant83/1 -> Switch30/1
  bit24/1 -> Switch30/2
  Switch30/1 -> Product23/1
  Saturation/1 -> Data Type Conversion/1
  Data Type Conversion/1 -> U32Out/1

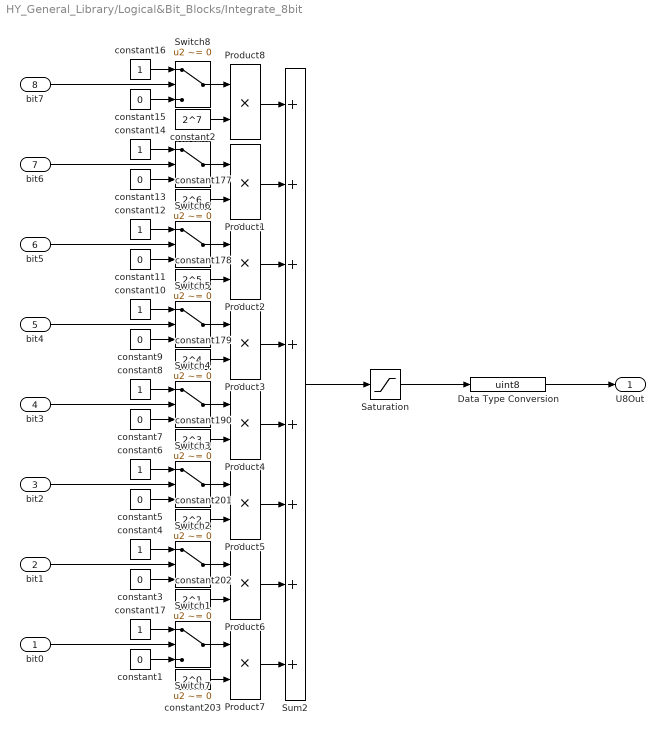
== system HY_General_Library/Logical&Bit_Blocks/Integrate_8bit ==
  bit0 : Inport
  bit1 : Inport  Port=2
  bit2 : Inport  Port=3
  bit3 : Inport  Port=4
  bit4 : Inport  Port=5
  bit5 : Inport  Port=6
  bit6 : Inport  Port=7
  bit7 : Inport  Port=8
  Data Type Conversion : DataTypeConversion  OutDataTypeStr=uint8
  Product{1..8} (8 alike) : Product  SaturateOnIntegerOverflow=on  InputSameDT=on  OutDataTypeStr=Inherit: Same as first input
  Saturation : Saturate  UpperLimit=255  LowerLimit=0
      settings: AttributesFormatString=%<LowerLimit> - %<UpperLimit>
  Sum2 : Sum  Inputs=8  SaturateOnIntegerOverflow=on  InputSameDT=on  OutDataTypeStr=Inherit: Same as first input
  Switch{1..8} (8 alike) : Switch  Criteria=u2 ~= 0  SaturateOnIntegerOverflow=on  InputSameDT=on
  constant{1,3,5,7,9,11,13,15} (8 alike) : Constant  Value=0  OutDataTypeStr=uint8
  constant{4,6,8,10,12,14,16..17} (8 alike) : Constant  OutDataTypeStr=uint8
  constant177 : Constant  Value=2^6  OutDataTypeStr=uint8
  constant178 : Constant  Value=2^5  OutDataTypeStr=uint8
  constant179 : Constant  Value=2^4  OutDataTypeStr=uint8
  constant190 : Constant  Value=2^3  OutDataTypeStr=uint8
  constant2 : Constant  Value=2^7  OutDataTypeStr=uint8
  constant201 : Constant  Value=2^2  OutDataTypeStr=uint8
  constant202 : Constant  Value=2^1  OutDataTypeStr=uint8
  constant203 : Constant  Value=2^0  OutDataTypeStr=uint8
  U8Out : Outport
  wires:
  Sum2/1 -> Saturation/1
  Product7/1 -> Sum2/8
  Product6/1 -> Sum2/7
  Product5/1 -> Sum2/6
  Product4/1 -> Sum2/5
  Product3/1 -> Sum2/4
  Product2/1 -> Sum2/3
  Product1/1 -> Sum2/2
  constant203/1 -> Product7/2
  constant202/1 -> Product6/2
  Switch1/1 -> Product6/1
  constant201/1 -> Product5/2
  Switch2/1 -> Product5/1
  constant190/1 -> Product4/2
  Switch3/1 -> Product4/1
  constant179/1 -> Product3/2
  Switch4/1 -> Product3/1
  constant178/1 -> Product2/2
  Switch5/1 -> Product2/1
  constant177/1 -> Product1/2
  Switch6/1 -> Product1/1
  Switch7/1 -> Product7/1
  Product8/1 -> Sum2/1
  constant2/1 -> Product8/2
  Switch8/1 -> Product8/1
  constant15/1 -> Switch8/3
  constant16/1 -> Switch8/1
  bit7/1 -> Switch8/2
  constant13/1 -> Switch6/3
  constant14/1 -> Switch6/1
  bit6/1 -> Switch6/2
  constant11/1 -> Switch5/3
  constant12/1 -> Switch5/1
  bit5/1 -> Switch5/2
  constant9/1 -> Switch4/3
  constant10/1 -> Switch4/1
  bit4/1 -> Switch4/2
  constant7/1 -> Switch3/3
  constant8/1 -> Switch3/1
  bit3/1 -> Switch3/2
  constant5/1 -> Switch2/3
  constant6/1 -> Switch2/1
  bit2/1 -> Switch2/2
  constant3/1 -> Switch1/3
  constant4/1 -> Switch1/1
  bit1/1 -> Switch1/2
  constant1/1 -> Switch7/3
  constant17/1 -> Switch7/1
  bit0/1 -> Switch7/2
  Saturation/1 -> Data Type Conversion/1
  Data Type Conversion/1 -> U8Out/1

== system HY_General_Library/Memory_Blocks/EdgeBi ==
  u : Inport  OutDataTypeStr=boolean
  Logical Operator : Logic  Operator=XOR  AllPortsSameDT=off  OutDataTypeStr=boolean
  Unit Delay2 : UnitDelay  SampleTime=-1
      settings: AttributesFormatString=<initial=%<x0>>
  y : Outport  OutDataTypeStr=boolean
  wires:
  u/1 -> Unit Delay2/1, Logical Operator/1
  Logical Operator/1 -> y/1
  Unit Delay2/1 -> Logical Operator/2

== system HY_General_Library/Memory_Blocks/EdgeFalling ==
  u : Inport  OutDataTypeStr=boolean
  Logical Operator : Logic  AllPortsSameDT=off  OutDataTypeStr=boolean
  Logical Operator2 : Logic  Operator=NOT  Inputs=1  AllPortsSameDT=off  OutDataTypeStr=boolean
  Unit Delay2 : UnitDelay  SampleTime=-1
      settings: AttributesFormatString=<initial=%<x0>>
  y : Outport  OutDataTypeStr=boolean
  wires:
  Unit Delay2/1 -> Logical Operator/2
  Logical Operator/1 -> y/1
  u/1 -> Unit Delay2/1, Logical Operator2/1
  Logical Operator2/1 -> Logical Operator/1

== system HY_General_Library/Memory_Blocks/EdgeRising ==
  u : Inport  OutDataTypeStr=boolean
  Logical Operator : Logic  AllPortsSameDT=off  OutDataTypeStr=boolean
  Logical Operator2 : Logic  Operator=NOT  Inputs=1  AllPortsSameDT=off  OutDataTypeStr=boolean
  Unit Delay2 : UnitDelay  SampleTime=-1
      settings: AttributesFormatString=<initial=%<x0>>
  y : Outport  OutDataTypeStr=boolean
  wires:
  u/1 -> Unit Delay2/1, Logical Operator/1
  Logical Operator/1 -> y/1
  Logical Operator2/1 -> Logical Operator/2
  Unit Delay2/1 -> Logical Operator2/1

== system HY_General_Library/Memory_Blocks/Mem ==
  u : Inport
  Hld : Inport  Port=2  OutDataTypeStr=boolean
  Switch1 : Switch  Criteria=u2 ~= 0  SaturateOnIntegerOverflow=on  InputSameDT=on
      settings: AttributesFormatString=|
      | %<Criteria>
      | threshold=%<threshold>
  UnitDelay : UnitDelay  SampleTime=-1
      settings: AttributesFormatString=<Initial=%<X0>>
  y : Outport
  wires:
  UnitDelay/1 -> Switch1/1
  Switch1/1 -> y/1, UnitDelay/1
  u/1 -> Switch1/3
  Hld/1 -> Switch1/2

== system HY_General_Library/Memory_Blocks/RS_FF ==
  S : Inport  OutDataTypeStr=boolean
  R : Inport  Port=2  OutDataTypeStr=boolean
  AND : Logic  OutDataTypeStr=boolean
  NOT : Logic  Operator=NOT  Inputs=1  OutDataTypeStr=boolean
  NOT2 : Logic  Operator=NOT  Inputs=1  OutDataTypeStr=boolean
  OR : Logic  Operator=OR  OutDataTypeStr=boolean
  Unit Delay : UnitDelay  InitialCondition=InitialValue  SampleTime=-1
      settings: AttributesFormatString=Init=%<X0>
  Q : Outport
  RQ : Outport  Port=2
  wires:
  AND/1 -> Q/1, NOT2/1, Unit Delay/1
  OR/1 -> AND/2
  NOT/1 -> AND/1
  R/1 -> NOT/1
  Unit Delay/1 -> OR/2
  S/1 -> OR/1
  NOT2/1 -> RQ/1

== system HY_General_Library/Memory_Blocks/RS_FF_IV ==
  S : Inport  OutDataTypeStr=boolean
  R : Inport  Port=2  OutDataTypeStr=boolean
  IV : Inport  Port=3  OutDataTypeStr=boolean
  AND : Logic  OutDataTypeStr=boolean
  Constant : Constant  Value=0  OutDataTypeStr=boolean
      settings: AttributesFormatString=%<OutDataTypeStr>
  NOT : Logic  Operator=NOT  Inputs=1  OutDataTypeStr=boolean
  NOT2 : Logic  Operator=NOT  Inputs=1  OutDataTypeStr=boolean
  OR : Logic  Operator=OR  OutDataTypeStr=boolean
  Switch : Switch  Criteria=u2 ~= 0  InputSameDT=on
      settings: AttributesFormatString=|
      | %<Criteria>
      | Threshold=%<Threshold>
  Unit Delay : UnitDelay  SampleTime=-1
      settings: AttributesFormatString=<initial=%<x0>>
  Unit Delay1 : UnitDelay  InitialCondition=1  SampleTime=-1
      settings: AttributesFormatString=<initial=%<x0>>
  Q : Outport
  RQ : Outport  Port=2
  wires:
  NOT2/1 -> RQ/1
  S/1 -> OR/1
  Unit Delay/1 -> Switch/3
  R/1 -> NOT/1
  NOT/1 -> AND/1
  OR/1 -> AND/2
  AND/1 -> Unit Delay/1, NOT2/1, Q/1
  Switch/1 -> OR/2
  IV/1 -> Switch/1
  Unit Delay1/1 -> Switch/2
  Constant/1 -> Unit Delay1/1

== system HY_General_Library/Memory_Blocks/RS_FF_IV_Neg ==
  S : Inport  OutDataTypeStr=boolean
  R : Inport  Port=2  OutDataTypeStr=boolean
  IV : Inport  Port=3  OutDataTypeStr=boolean
  AND : Logic  OutDataTypeStr=boolean
  Constant : Constant  Value=0  OutDataTypeStr=boolean
      settings: AttributesFormatString=%<OutDataTypeStr>
  NOT : Logic  Operator=NOT  Inputs=1  OutDataTypeStr=boolean
  NOT2 : Logic  Operator=NOT  Inputs=1  OutDataTypeStr=boolean
  OR : Logic  Operator=OR  OutDataTypeStr=boolean
  Switch : Switch  Criteria=u2 ~= 0  InputSameDT=on
      settings: AttributesFormatString=|
      | %<Criteria>
      | Threshold=%<Threshold>
  Unit Delay : UnitDelay  SampleTime=-1
      settings: AttributesFormatString=<initial=%<x0>>
  Unit Delay1 : UnitDelay  InitialCondition=1  SampleTime=-1
      settings: AttributesFormatString=<initial=%<x0>>
  RQ : Outport
  wires:
  Constant/1 -> Unit Delay1/1
  Unit Delay1/1 -> Switch/2
  IV/1 -> Switch/1
  Switch/1 -> OR/2
  AND/1 -> Unit Delay/1, NOT2/1
  OR/1 -> AND/2
  NOT/1 -> AND/1
  R/1 -> NOT/1
  Unit Delay/1 -> Switch/3
  S/1 -> OR/1
  NOT2/1 -> RQ/1

== system HY_General_Library/Memory_Blocks/RS_FF_IV_Pos ==
  S : Inport  OutDataTypeStr=boolean
  R : Inport  Port=2  OutDataTypeStr=boolean
  IV : Inport  Port=3  OutDataTypeStr=boolean
  AND : Logic  OutDataTypeStr=boolean
  Constant : Constant  Value=0  OutDataTypeStr=boolean
      settings: AttributesFormatString=%<OutDataTypeStr>
  NOT : Logic  Operator=NOT  Inputs=1  OutDataTypeStr=boolean
  OR : Logic  Operator=OR  OutDataTypeStr=boolean
  Switch : Switch  Criteria=u2 ~= 0  InputSameDT=on
      settings: AttributesFormatString=|
      | %<Criteria>
      | Threshold=%<Threshold>
  Unit Delay : UnitDelay  SampleTime=-1
      settings: AttributesFormatString=<initial=%<x0>>
  Unit Delay1 : UnitDelay  InitialCondition=1  SampleTime=-1
      settings: AttributesFormatString=<initial=%<x0>>
  Q : Outport
  wires:
  Constant/1 -> Unit Delay1/1
  Unit Delay1/1 -> Switch/2
  IV/1 -> Switch/1
  Switch/1 -> OR/2
  AND/1 -> Q/1, Unit Delay/1
  OR/1 -> AND/2
  NOT/1 -> AND/1
  R/1 -> NOT/1
  Unit Delay/1 -> Switch/3
  S/1 -> OR/1

== system HY_General_Library/Memory_Blocks/RS_FF_Neg ==
  S : Inport  OutDataTypeStr=boolean
  R : Inport  Port=2  OutDataTypeStr=boolean
  AND : Logic  OutDataTypeStr=boolean
  NOT : Logic  Operator=NOT  Inputs=1  OutDataTypeStr=boolean
  NOT1 : Logic  Operator=NOT  Inputs=1  OutDataTypeStr=boolean
  OR : Logic  Operator=OR  OutDataTypeStr=boolean
  Unit Delay : UnitDelay  InitialCondition=InitialValue  SampleTime=-1
      settings: AttributesFormatString=Init=%<X0>
  RQ : Outport
  wires:
  S/1 -> OR/1
  Unit Delay/1 -> OR/2
  AND/1 -> NOT1/1, Unit Delay/1
  R/1 -> NOT/1
  NOT/1 -> AND/1
  OR/1 -> AND/2
  NOT1/1 -> RQ/1

== system HY_General_Library/Memory_Blocks/RS_FF_Pos ==
  S : Inport  OutDataTypeStr=boolean
  R : Inport  Port=2  OutDataTypeStr=boolean
  AND : Logic  OutDataTypeStr=boolean
  NOT : Logic  Operator=NOT  Inputs=1  OutDataTypeStr=boolean
  OR : Logic  Operator=OR  OutDataTypeStr=boolean
  Unit Delay : UnitDelay  InitialCondition=InitialValue  SampleTime=-1
      settings: AttributesFormatString=Init=%<X0>
  Q : Outport
  wires:
  OR/1 -> AND/2
  NOT/1 -> AND/1
  R/1 -> NOT/1
  AND/1 -> Unit Delay/1, Q/1
  Unit Delay/1 -> OR/2
  S/1 -> OR/1
